simulink model "Model"  (R2022b)
settings: Solver=VariableStepAuto  StartTime=0.0  StopTime=10.0  RelTol=1e-3
settings Model: Creator=Abdelrhman Shaban  LastModifiedBy=Abdelrhman Shaban

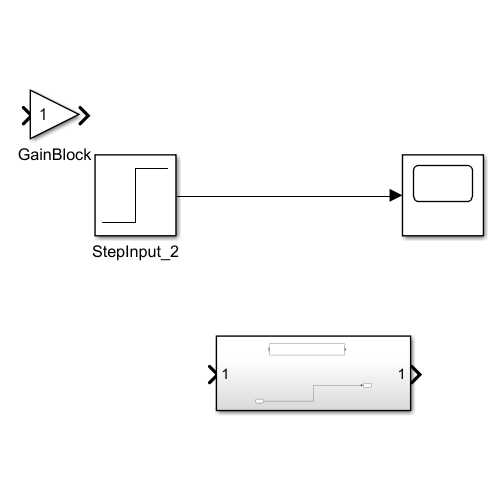
[thumbnail: Simulink's stored preview of the top-level diagram]
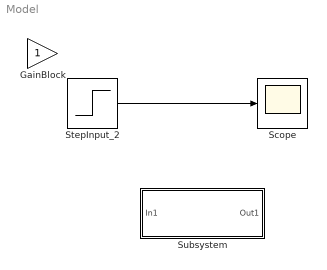
== system Model ==
  GainBlock : Gain
  Scope : Scope
  StepInput_2 : Step
  Subsystem : Subsystem
  wires:
  StepInput_2/1 -> Scope/1

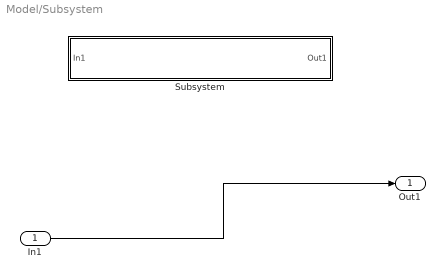
== system Model/Subsystem ==
  In1 : Inport
  Subsystem : Subsystem
  Out1 : Outport
  wires:
  In1/1 -> Out1/1

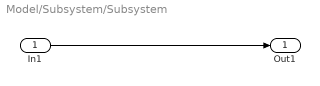
== system Model/Subsystem/Subsystem ==
  In1 : Inport
  Out1 : Outport
  wires:
  In1/1 -> Out1/1
